simulink model "Paper1_SM"  (R2020b)
settings: Solver=ode4  StartTime=0.0  StopTime=40  FixedStep=0.01  RelTol=1e-3
settings Model: Creator=zhiyao  LastModifiedBy=zhiyao
settings DataIOCC: ReturnWorkspaceOutputs=off

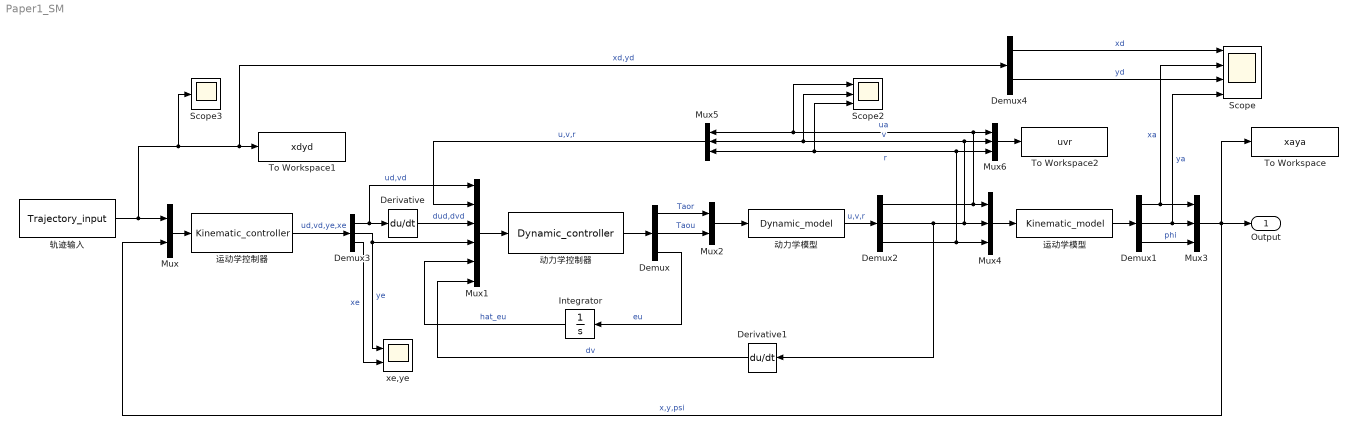
== system Paper1_SM ==
  Demux : Demux  Outputs=3
  Demux1 : Demux  Outputs=3
  Demux2 : Demux  Outputs=3
  Demux3 : Demux  Outputs=[2 1 1]
  Demux4 : Demux  Outputs=2
  Derivative : Derivative
  Derivative1 : Derivative
  Integrator : Integrator
  Mux : Mux  Inputs=2
  Mux1 : Mux  Inputs=6
  Mux2 : Mux  Inputs=2
  Mux{3..6} (4 alike) : Mux  Inputs=3
  Scope : Scope  NumInputPorts=4
  Scope2 : Scope  NumInputPorts=3
  Scope3 : Scope
  To Workspace : ToWorkspace  VariableName=xaya  SampleTime=-1
  To Workspace1 : ToWorkspace  VariableName=xdyd  SampleTime=-1
  To Workspace2 : ToWorkspace  VariableName=uvr  SampleTime=-1
  xe,ye : Scope  NumInputPorts=2
  动力学控制器 : S-Function  FunctionName=Dynamic_controller  Parameters=pa  SFunctionDeploymentMode=off  EnableBusSupport=off
  动力学模型 : S-Function  FunctionName=Dynamic_model  Parameters=pa  SFunctionDeploymentMode=off  EnableBusSupport=off
  轨迹输入 : S-Function  FunctionName=Trajectory_input  Parameters=pa  SFunctionDeploymentMode=off  EnableBusSupport=off
  运动学控制器 : S-Function  FunctionName=Kinematic_controller  Parameters=pa  SFunctionDeploymentMode=off  EnableBusSupport=off
  运动学模型 : S-Function  FunctionName=Kinematic_model  SFunctionDeploymentMode=off  EnableBusSupport=off
  Output : Outport
  wires:
  Mux/1 -> 运动学控制器/1
  Mux1/1 -> 动力学控制器/1
  Derivative/1 -> Mux1/3  "dud,dvd"
  Demux/1 -> Mux2/1  "Taor"
  Demux/2 -> Mux2/2  "Taou"
  Mux2/1 -> 动力学模型/1
  运动学模型/1 -> Demux1/1
  Demux1/2 -> Scope/4, Mux3/2  "ya"
  Demux1/1 -> Mux3/1, Scope/2  "xa"
  Mux3/1 -> To Workspace/1, Mux/2, Output/1  "x,y,psi"
  Demux1/3 -> Mux3/3  "phi"
  Demux/3 -> Integrator/1  "eu"
  Integrator/1 -> Mux1/5  "hat_eu"
  轨迹输入/1 -> Scope3/1, Demux4/1, To Workspace1/1, Mux/1  "xd,yd"
  动力学模型/1 -> Demux2/1  "u,v,r"
  Mux4/1 -> 运动学模型/1
  Demux2/1 -> Mux4/1, Mux6/1, Scope2/1, Mux5/1  "ua"
  Demux2/2 -> Derivative1/1, Mux4/2, Mux6/2, Scope2/2, Mux5/2  "v"
  Demux2/3 -> Mux4/3, Mux6/3, Scope2/3, Mux5/3  "r"
  Mux5/1 -> Mux1/2  "u,v,r"
  Derivative1/1 -> Mux1/6  "dv"
  运动学控制器/1 -> Demux3/1  "ud,vd,ye,xe"
  Demux3/1 -> Mux1/1, Derivative/1  "ud,vd"
  Demux3/2 -> Mux1/4, xe,ye/1  "ye"
  动力学控制器/1 -> Demux/1
  Demux4/1 -> Scope/1  "xd"
  Demux4/2 -> Scope/3  "yd"
  Demux3/3 -> xe,ye/2  "xe"
  Mux6/1 -> To Workspace2/1
